simulink model "Position"  (R2015a)
settings: Solver=ode2  StartTime=0.0  StopTime=10.0  FixedStep=tc  RelTol=1e-3
InitFcn:
  | Parameters
values from neighbouring files (symbols this model uses):
  pitchMax = pi/6    (= 0.523598775598)    [Parameters.m]
  rollMax = pi/6    (= 0.523598775598)    [Parameters.m]
undefined symbols (not defined in the file or in its folder): KD, KI, KN, KP
libraries: simulink x2
settings Model: Creator=pela  LastModifiedBy=Mattia
settings HardwareCC: ProdLargestAtomicInteger=Long  ProdLargestAtomicFloat=Double  ProdEndianess=LittleEndian  ProdHWDeviceType=ARM Compatible->ARM Cortex
settings RTWCC: GenCodeOnly=on  GenerateReport=on  Toolchain=Microsoft Visual C++ 2013 v12.0 | nmake (64-bit Windows)  BuildConfiguration=Faster Runs  LaunchReport=on  TargetLang=C++
settings GRTTargetCC: MatFileLogging=off  MultiInstanceERTCode=on  CodeInterfacePackaging=C++ class  SupportNonFinite=off

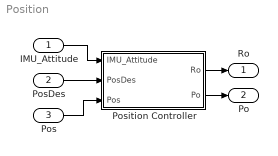
== system Position ==
  IMU_Attitude : Inport
  PosDes : Inport  Port=2
  Pos : Inport  Port=3
  Position Controller : Subsystem
  Ro : Outport
  Po : Outport  Port=2
  wires:
  Position Controller/1(Ro) -> Ro/1
  Position Controller/2(Po) -> Po/1
  Pos/1 -> Position Controller/3(Pos)
  PosDes/1 -> Position Controller/2(PosDes)
  IMU_Attitude/1 -> Position Controller/1(IMU_Attitude)

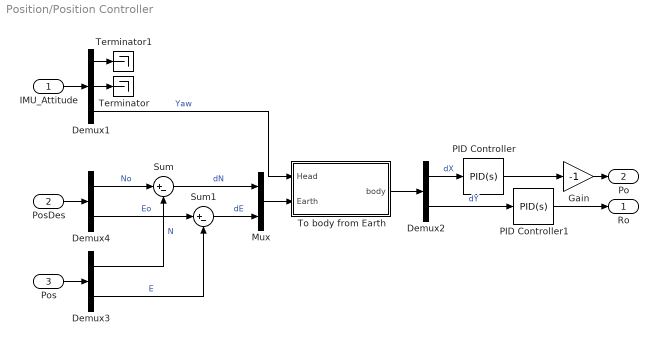
== system Position/Position Controller ==
  IMU_Attitude : Inport
  PosDes : Inport  Port=2
  Pos : Inport  Port=3
  Demux1 : Demux  Outputs=3
  Demux2 : Demux  Outputs=2
  Demux3 : Demux  Outputs=2
  Demux4 : Demux  Outputs=2
  Gain : Gain  Gain=-1
  Mux : Mux  Inputs=2
  PID Controller : simulink/Continuous/PID Controller  Controller=PID  TimeDomain=Continuous-time  SampleTime=-1  IntegratorMethod=Forward Euler  FilterMethod=Forward Euler  Form=Parallel  UseFilter=on  ControllerParametersSource=internal  P=KP  I=KI  D=KD  N=KN  InitialConditionSource=internal  InitialConditionForIntegrator=0  InitialConditionForFilter=0  ExternalReset=none  LimitOutput=on  UpperSaturationLimit=pitchMax  LowerSaturationLimit=-pitchMax  LinearizeAsGain=on  AntiWindupMode=none  Kb=1  TrackingMode=off  Kt=1  PParamMin=[]  PParamMax=[]  IParamMin=[]  IParamMax=[]  DParamMin=[]  DParamMax=[]  NParamMin=[]  NParamMax=[]  KbParamMin=[]  KbParamMax=[]  KtParamMin=[]  KtParamMax=[]  POutMin=[]  POutMax=[]  IOutMin=[]  IOutMax=[]  DOutMin=[]  DOutMax=[]  NOutMin=[]  NOutMax=[]  KbOutMin=[]  KbOutMax=[]  KtOutMin=[]  KtOutMax=[]  IntegratorOutMin=[]  IntegratorOutMax=[]  FilterOutMin=[]  FilterOutMax=[]  SumOutMin=[]  SumOutMax=[]  SumI1OutMin=[]  SumI1OutMax=[]  SumI2OutMin=[]  SumI2OutMax=[]  SumI3OutMin=[]  SumI3OutMax=[]  SumDOutMin=[]  SumDOutMax=[]  SaturationOutMin=[]  SaturationOutMax=[]  IntegratorContinuousStateAttributes=''  IntegratorStateMustResolveToSignalObject=off  IntegratorRTWStateStorageClass=Auto  FilterContinuousStateAttributes=''  FilterStateMustResolveToSignalObject=off  FilterRTWStateStorageClass=Auto  DifferentiatorICPrevScaledInput=0  DifferentiatorOutMin=[]  DifferentiatorOutMax=[]
  PID Controller1 : simulink/Continuous/PID Controller  Controller=PID  TimeDomain=Continuous-time  SampleTime=-1  IntegratorMethod=Forward Euler  FilterMethod=Forward Euler  Form=Parallel  UseFilter=on  ControllerParametersSource=internal  P=KP  I=KI  D=KD  N=KN  InitialConditionSource=internal  InitialConditionForIntegrator=0  InitialConditionForFilter=0  ExternalReset=none  LimitOutput=on  UpperSaturationLimit=rollMax  LowerSaturationLimit=-rollMax  LinearizeAsGain=on  AntiWindupMode=none  Kb=1  TrackingMode=off  Kt=1  PParamMin=[]  PParamMax=[]  IParamMin=[]  IParamMax=[]  DParamMin=[]  DParamMax=[]  NParamMin=[]  NParamMax=[]  KbParamMin=[]  KbParamMax=[]  KtParamMin=[]  KtParamMax=[]  POutMin=[]  POutMax=[]  IOutMin=[]  IOutMax=[]  DOutMin=[]  DOutMax=[]  NOutMin=[]  NOutMax=[]  KbOutMin=[]  KbOutMax=[]  KtOutMin=[]  KtOutMax=[]  IntegratorOutMin=[]  IntegratorOutMax=[]  FilterOutMin=[]  FilterOutMax=[]  SumOutMin=[]  SumOutMax=[]  SumI1OutMin=[]  SumI1OutMax=[]  SumI2OutMin=[]  SumI2OutMax=[]  SumI3OutMin=[]  SumI3OutMax=[]  SumDOutMin=[]  SumDOutMax=[]  SaturationOutMin=[]  SaturationOutMax=[]  IntegratorContinuousStateAttributes=''  IntegratorStateMustResolveToSignalObject=off  IntegratorRTWStateStorageClass=Auto  FilterContinuousStateAttributes=''  FilterStateMustResolveToSignalObject=off  FilterRTWStateStorageClass=Auto  DifferentiatorICPrevScaledInput=0  DifferentiatorOutMin=[]  DifferentiatorOutMax=[]
  Sum : Sum  Inputs=|+-
  Sum1 : Sum  Inputs=|+-
  Terminator : Terminator
  Terminator1 : Terminator
  To body from Earth : MATLAB Function  TreatAsAtomicUnit=on
  Ro : Outport
  Po : Outport  Port=2
  wires:
  IMU_Attitude/1 -> Demux1/1
  Demux1/1 -> Terminator1/1
  Demux1/2 -> Terminator/1
  PID Controller1/1 -> Ro/1
  PID Controller/1 -> Gain/1
  Gain/1 -> Po/1
  Demux2/1 -> PID Controller/1  "dX"
  Demux2/2 -> PID Controller1/1  "dY"
  To body from Earth/1(body) -> Demux2/1
  Pos/1 -> Demux3/1
  Demux3/1 -> Sum/2  "N"
  Demux3/2 -> Sum1/2  "E"
  Sum1/1 -> Mux/2  "dE"
  Sum/1 -> Mux/1  "dN"
  Mux/1 -> To body from Earth/2(Earth)
  Demux1/3 -> To body from Earth/1(Head)  "Yaw"
  Demux4/1 -> Sum/1  "No"
  Demux4/2 -> Sum1/1  "Eo"
  PosDes/1 -> Demux4/1

== matlab function Position/Position Controller/To body from Earth ==
  data: Head input; body output; Earth input
function body = Earth(Head, Earth)
%#codegen
psi = Head;

Spsi = sin(psi);
Cpsi = cos(psi);

TBE = [ Cpsi Spsi ;
       -Spsi Cpsi];

body = TBE* Earth;
